simulink model "TxArray"  (R2021b)
settings: Solver=FixedStepDiscrete  StartTime=0.0  StopTime=50  FixedStep=0.01  RelTol=1e-3  EnableMultiTasking=on
libraries: raspberrypiNetworklib x4, realtime_pacer_lib x1
settings Model: SnapshotBufferSize=50  PacingRate=1000  Creator=Blade  LastModifiedBy=Blade
settings SolverCC: PositivePriorityOrder=on

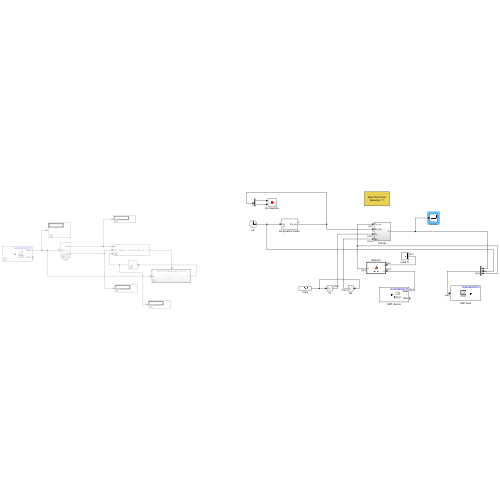
[thumbnail: Simulink's stored preview of the top-level diagram]
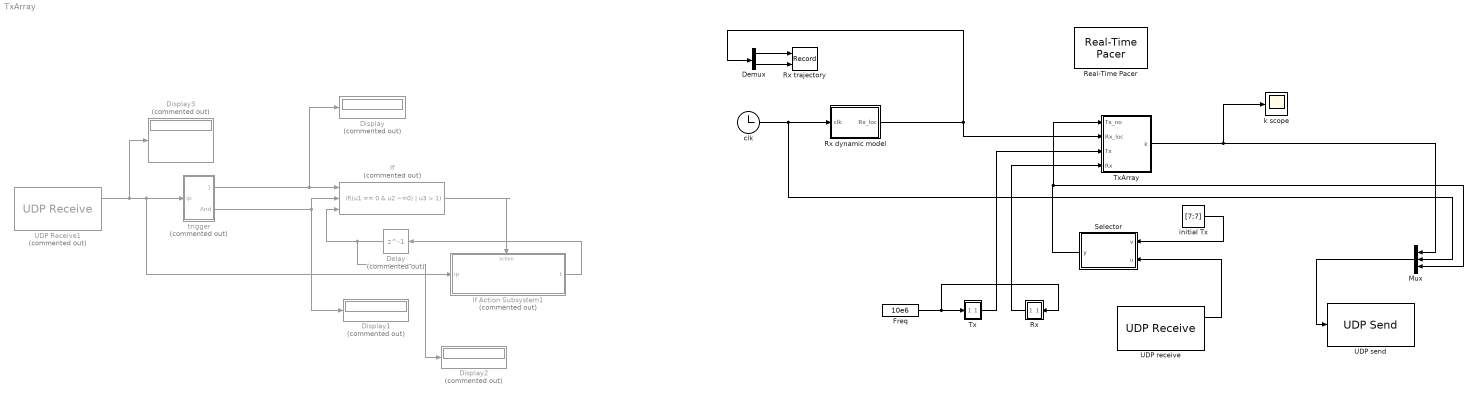
== system TxArray ==
  Delay : Delay  Commented=on  DelayLength=1  InitialCondition=0
  Demux : Demux  Outputs=2
  Display{,1..3} (4 alike) : Display  Commented=on
  Freq : Constant  Value=10e6
  If : If  Commented=on  NumInputs=3  IfExpression=(u1 == 0 & u2 ~=0) | u3 > 1  ShowElse=off
  If Action Subsystem1 : Subsystem  Commented=on  TreatAsAtomicUnit=on
  Mux : Mux  Inputs=3
  Real-Time Pacer : realtime_pacer_lib/Real-Time Pacer  simTimePerRealTime=1
      settings: SourceProductName=Real-Time Pacer
  Rx : Subsystem  mask{dout=1/3*100e-3, phi=0.15, s=800e-6, w=1200e-6, CP=0, SR=0.01}
      mask prompts: dout "out diameter"; phi "fillfact"; s "track spacing"; w "track width"; CP "parasitic capacitance"; SR "source resistance"
      mask TypeOptions dout: Constant1/Value
      mask TypeOptions phi: Constant2/Value
      mask TypeOptions s: Constant3/Value
      mask TypeOptions w: Constant4/Value
      mask TypeOptions CP: Constant6/Value
      mask TypeOptions SR: Constant7/Value
  "Rx dynamic model " : Subsystem  mask{initx=1/2*100e-3*(7+1), inity=1/2*100e-3*(7+1), v_min=[0.01,0.01], v_max=[0.02,0.02]}
      mask prompts: initx "Rx initial x"; inity "Rx initial y"; v_min "Rx min speed"; v_max "Rx max speed"
      mask TypeOptions initx: Delay1/InitialCondition
      mask TypeOptions inity: Delay2/InitialCondition
      mask TypeOptions v_min: Constant/Value
      mask TypeOptions v_max: Constant1/Value
  Rx trajectory : Record  RecordToWorkspace=on  FileSettingsInternal="{\"entries\":[{\"content\":{\"excelSettings\":{\"content\":{},\"type\":\"Streamout.ExcelSettings\"}},\"type\":\"Streamout.FileSettingStorage\",\"uuid\":\"31a4ec05-c512-48d1-876e-5766672d7d43\"}],\"packageUris\":[\"http://schema.mathworks.com/mf0/streamout_blocks/R2020a\"],\"version\":\"1.0\"}"  Layout=[1 1]  SignalsInternal="{\"entries\":[{\"content\":{\"signals\":[{\"content\":{\"blockPath\":[\"TxArray/Rx trajectory\"],\"channel\":[],\"dimensions\":[1],\"domain\":\"TxArray/Rx trajectory\",\"lineColor\":\"#a2142f\",\"plots\":[1],\"port\":1,\"sid\":[\"\"],\"signalID\":51290,\"signalName\":\"Demux:1\"},\"type\":\"RecordBlkView.Signal\",\"uuid\":\"0aae7323-a21c-435c-a499-c26e652a0b80\"},{\"content\":{\"blockPath\":[\"TxArray/Rx trajectory\"],\"channel\":[],\"dimensions\":[1],\"domain\":\"TxArray/Rx trajectory\",\"lineColor\":\"#139fff\",\"plots\":[1],\"port\":2,\"sid\":[\"\"],\"signalID\":51294,\"signalName\":\"Demux:2\"},\"type\":\"RecordBlkView.Signal\",\"uuid\":\"970d65ca-2c0e-4b4c-8729-1a3121c9315b\"}]},\"type\":\"RecordBlkView.InputSignals\",\"uuid\":\"1676dd2b-c950-4d6b-bdb0-46605d271428\"}],\"packageUris\":[\"http://schema.mathworks.com/mf0/streamout_blocks/R2020a\"],\"version\":\"1.0\"}"  VisualizationBindings="{\"xyplotplugin\":{\"info\":[{\"series\":[{\"bindingParametersList\":[{\"parameter\":\"X-Axis\",\"signalID\":51290,\"signalName\":\"Demux:1\"},{\"parameter\":\"Y-Axis\",\"signalID\":51294,\"signalName\":\"Demux:2\"}],\"seriesID\":44186}],\"subplotID\":1}]}}"  CompatibilityTag=XY
  Selector : MATLAB Function  TreatAsAtomicUnit=on
  Tx : Subsystem  mask{dout=100e-3, phi=0.25, s=3*2500e-6, w=2500e-6, CP=0, SR=0.01}
      mask prompts: dout "out diameter"; phi "fillfact"; s "track spacing"; w "track width"; CP "parasitic capacitance"; SR "source resistance"
      mask TypeOptions dout: Constant1/Value
      mask TypeOptions phi: Constant2/Value
      mask TypeOptions s: Constant3/Value
      mask TypeOptions w: Constant4/Value
      mask TypeOptions CP: Constant6/Value
      mask TypeOptions SR: Constant7/Value
  TxArray : Subsystem
  UDP Receive1 : raspberrypiNetworklib/UDP Receive  Commented=on  localURL='0.0.0.0'  localPort=1000  remoteURL='0.0.0.0'  remotePort=-1  recvBufferSize=8192  signalDatatype=double  dims=4  isVarSize=off  showBlockingTime=off  blockingTime=0  sampletime=-1  blockPlatform=Raspberry Pi
      settings: SourceProductBaseCode=RASPPI
  UDP receive : raspberrypiNetworklib/UDP Receive  localURL='0.0.0.0'  localPort=2000  remoteURL='0.0.0.0'  remotePort=-1  recvBufferSize=8192  signalDatatype=double  dims=2  isVarSize=off  showBlockingTime=off  blockingTime=0  sampletime=-1  blockPlatform=Raspberry Pi
      settings: SourceProductBaseCode=RASPPI
  UDP send : raspberrypiNetworklib/UDP Send  remoteURL='172.20.10.3'  remotePort=1000  localURL='0.0.0.0'  localPortSource=Automatically determine  localPort=-1  sampletime=-1  blockPlatform=Raspberry Pi  separateLengthPort=0
      settings: SourceProductBaseCode=RASPPI
  clk : Clock
  initial Tx : Constant  Value=[7;7]  VectorParams1D=off
  k scope : Scope
  trigger : Subsystem  Commented=on
  wires:
  Rx/1(Out1) -> TxArray/4(Rx)
  "Rx dynamic model "/1(Rx_loc) -> TxArray/2(Rx_loc), Demux/1
  Demux/1 -> Rx trajectory/1
  Freq/1 -> Rx/1(In1), Tx/1(In1)
  Demux/2 -> Rx trajectory/2
  Tx/1(Out1) -> TxArray/3(Tx)
  clk/1 -> Mux/2, "Rx dynamic model "/1(clk)
  TxArray/1(k) -> k scope/1, Mux/1
  Selector/1(y) -> Mux/3, TxArray/1(Tx_no)
  UDP receive/1 -> Selector/2(u)
  Mux/1 -> UDP send/1
  initial Tx/1 -> Selector/1(v)
  If/1 -> If Action Subsystem1/Action
  If Action Subsystem1/1(t) -> Delay/1
  trigger/1(mod) -> If/1, Display/1
  Delay/1 -> Display2/1, If/3
  trigger/2(And) -> If/2, Display1/1
  UDP Receive1/1 -> Display3/1, If Action Subsystem1/1(ip), trigger/1(ip)

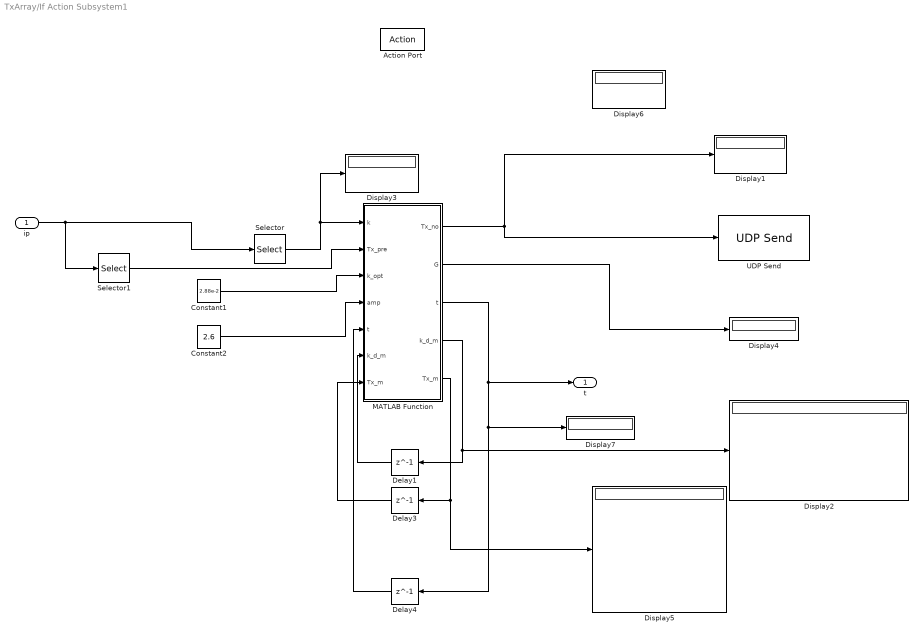
== system TxArray/If Action Subsystem1 ==
  ip : Inport
  Action Port : ActionPort  ActionPortLabel=if((u1 == 0 & u2 ~=0) | u3 > 1)
  Constant1 : Constant  Value=2.88e-2
  Constant2 : Constant  Value=2.6
  Delay1 : Delay  DelayLength=1  InitialCondition=zeros(2,3)
  Delay3 : Delay  DelayLength=1  InitialCondition=zeros(8,2)
  Delay4 : Delay  DelayLength=1  InitialCondition=0
  Display{1..7} (7 alike) : Display
  MATLAB Function : MATLAB Function  TreatAsAtomicUnit=on
  Selector : Selector  InputPortWidth=4  IndexOptions=Index vector (dialog)  Indices=1  OutputSizes=1
  Selector1 : Selector  InputPortWidth=4  IndexOptions=Index vector (dialog)  Indices=[3;4]  OutputSizes=1
  UDP Send : raspberrypiNetworklib/UDP Send  remoteURL='172.20.10.2'  remotePort=2000  localURL='0.0.0.0'  localPortSource=Automatically determine  localPort=-1  sampletime=-1  blockPlatform=Raspberry Pi  separateLengthPort=0
      settings: SourceProductBaseCode=RASPPI
  t : Outport
  wires:
  Delay4/1 -> MATLAB Function/5("t ")
  Constant2/1 -> MATLAB Function/4(amp)
  ip/1 -> Selector1/1, Selector/1
  Constant1/1 -> MATLAB Function/3(k_opt)
  MATLAB Function/1(Tx_no) -> UDP Send/1, Display1/1
  MATLAB Function/3(t) -> Display7/1, Delay4/1, t/1
  MATLAB Function/4(k_d_m) -> Delay1/1, Display2/1
  MATLAB Function/5(Tx_m) -> Display5/1, Delay3/1
  Selector/1 -> Display3/1, MATLAB Function/1(k)
  Delay1/1 -> MATLAB Function/6("k_d_m ")
  MATLAB Function/2(G) -> Display4/1
  Delay3/1 -> MATLAB Function/7("Tx_m ")
  Selector1/1 -> MATLAB Function/2(Tx_pre)

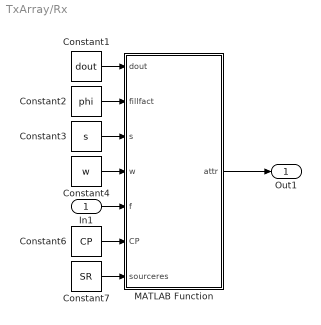
== system TxArray/Rx ==
  In1 : Inport
  Constant1 : Constant  Value=dout
  Constant2 : Constant  Value=phi
  Constant3 : Constant  Value=s
  Constant4 : Constant  Value=w
  Constant6 : Constant  Value=CP
  Constant7 : Constant  Value=SR
  MATLAB Function : MATLAB Function  TreatAsAtomicUnit=on
  Out1 : Outport
  wires:
  MATLAB Function/1(attr) -> Out1/1
  Constant7/1 -> MATLAB Function/7(sourceres)
  Constant1/1 -> MATLAB Function/1(dout)
  Constant2/1 -> MATLAB Function/2(fillfact)
  Constant3/1 -> MATLAB Function/3(s)
  Constant4/1 -> MATLAB Function/4(w)
  In1/1 -> MATLAB Function/5(f)
  Constant6/1 -> MATLAB Function/6(CP)

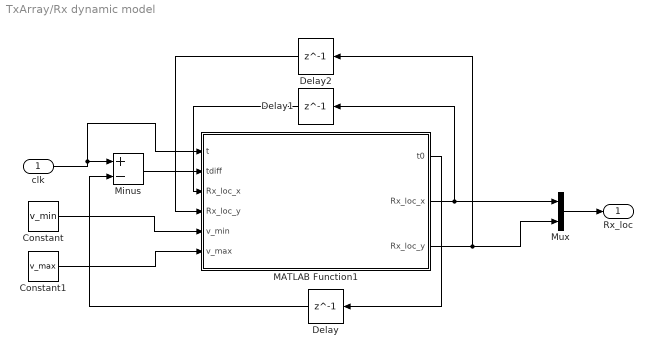
== system TxArray/Rx dynamic model  ==
  clk : Inport
  Constant : Constant  Value=v_min  VectorParams1D=off
  Constant1 : Constant  Value=v_max  VectorParams1D=off
  Delay : Delay  DelayLength=1  InitialCondition=0
  Delay1 : Delay  DelayLength=1  InitialCondition=initx
  Delay2 : Delay  DelayLength=1  InitialCondition=inity
  MATLAB Function1 : MATLAB Function  TreatAsAtomicUnit=on
  Minus : Sum  Inputs=+-
  Mux : Mux  Inputs=2
  Rx_loc : Outport
  wires:
  MATLAB Function1/3(Rx_loc_y) -> Delay2/1, Mux/2
  Delay/1 -> Minus/2
  clk/1 -> MATLAB Function1/1(t), Minus/1
  Delay2/1 -> MATLAB Function1/4("Rx_loc_y ")
  MATLAB Function1/1(t0) -> Delay/1
  Minus/1 -> MATLAB Function1/2(tdiff)
  Delay1/1 -> MATLAB Function1/3("Rx_loc_x ")
  MATLAB Function1/2(Rx_loc_x) -> Delay1/1, Mux/1
  Mux/1 -> Rx_loc/1
  Constant/1 -> MATLAB Function1/5(v_min)
  Constant1/1 -> MATLAB Function1/6(v_max)

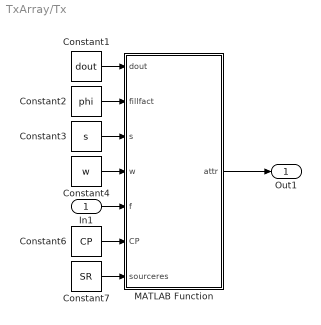
== system TxArray/Tx ==
  In1 : Inport
  Constant1 : Constant  Value=dout
  Constant2 : Constant  Value=phi
  Constant3 : Constant  Value=s
  Constant4 : Constant  Value=w
  Constant6 : Constant  Value=CP
  Constant7 : Constant  Value=SR
  MATLAB Function : MATLAB Function  TreatAsAtomicUnit=on
  Out1 : Outport
  wires:
  MATLAB Function/1(attr) -> Out1/1
  Constant7/1 -> MATLAB Function/7(sourceres)
  Constant1/1 -> MATLAB Function/1(dout)
  Constant2/1 -> MATLAB Function/2(fillfact)
  Constant3/1 -> MATLAB Function/3(s)
  Constant4/1 -> MATLAB Function/4(w)
  In1/1 -> MATLAB Function/5(f)
  Constant6/1 -> MATLAB Function/6(CP)

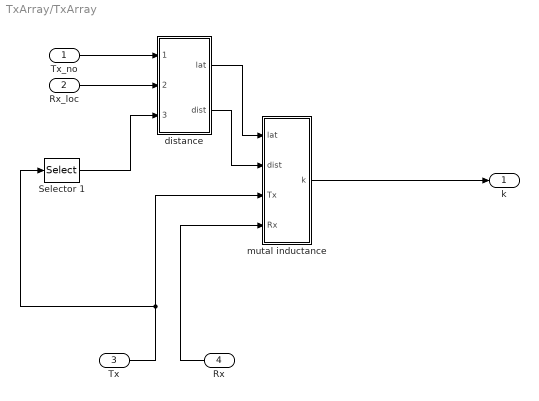
== system TxArray/TxArray ==
  Tx_no : Inport
  Rx_loc : Inport  Port=2
  Tx : Inport  Port=3
  Rx : Inport  Port=4
  " mutal inductance" : Subsystem
  Selector 1 : Selector  InputPortWidth=14  IndexOptions=Index vector (dialog)  Indices=1  OutputSizes=1
  distance : Subsystem
  k : Outport
  wires:
  Tx/1 -> Selector 1/1, " mutal inductance"/3(Tx)
  distance/1(lat) -> " mutal inductance"/1(lat)
  Rx/1 -> " mutal inductance"/4(Rx)
  Tx_no/1 -> distance/1(Tx_no)
  Rx_loc/1 -> distance/2(Rx_loc)
  Selector 1/1 -> distance/3(Tx_dia)
  " mutal inductance"/1(k) -> k/1
  distance/2(dist) -> " mutal inductance"/2(dist)

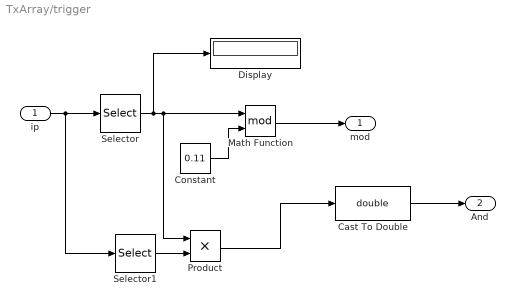
== system TxArray/trigger ==
  ip : Inport
  Cast To Double : DataTypeConversion  OutDataTypeStr=double
  Constant : Constant  Value=0.11
  Display : Display
  Math Function : Math  Operator=mod  SaturateOnIntegerOverflow=on
  Product : Product
  Selector : Selector  InputPortWidth=4  IndexOptions=Index vector (dialog)  Indices=2  OutputSizes=1
  Selector1 : Selector  InputPortWidth=4  IndexOptions=Index vector (dialog)  Indices=1  OutputSizes=1
  mod : Outport
  And : Outport  Port=2
  wires:
  Constant/1 -> Math Function/2
  Selector/1 -> Display/1, Product/1, Math Function/1
  ip/1 -> Selector1/1, Selector/1
  Math Function/1 -> mod/1
  Product/1 -> Cast To Double/1
  Selector1/1 -> Product/2
  Cast To Double/1 -> And/1

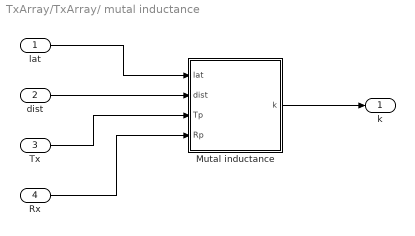
== system TxArray/TxArray/ mutal inductance ==
  lat : Inport
  dist : Inport  Port=2
  Tx : Inport  Port=3
  Rx : Inport  Port=4
  Mutal inductance : MATLAB Function  TreatAsAtomicUnit=on
  k : Outport
  wires:
  lat/1 -> Mutal inductance/1(lat)
  dist/1 -> Mutal inductance/2(dist)
  Tx/1 -> Mutal inductance/3(Tp)
  Rx/1 -> Mutal inductance/4(Rp)
  Mutal inductance/1(k) -> k/1

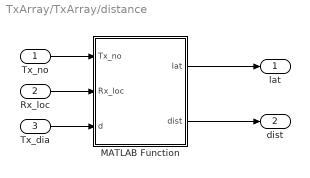
== system TxArray/TxArray/distance ==
  Tx_no : Inport
  Rx_loc : Inport  Port=2
  Tx_dia : Inport  Port=3
  MATLAB Function : MATLAB Function  TreatAsAtomicUnit=on
  lat : Outport
  dist : Outport  Port=2
  wires:
  Tx_dia/1 -> MATLAB Function/3(d)
  Tx_no/1 -> MATLAB Function/1(Tx_no)
  Rx_loc/1 -> MATLAB Function/2(Rx_loc)
  MATLAB Function/1(lat) -> lat/1
  MATLAB Function/2(dist) -> dist/1

== matlab function TxArray/distance/MATLAB Function ==
  data: Tx_no input; Rx_loc input; d input; lat output; dist output
function [lat, dist] = distance(Tx_no, Rx_loc, d)

coder.extrinsic('lat_dist');
coder.extrinsic('vertical_dist');


lat = 0;
dist = 0;

lat = lat_dist(Tx_no, Rx_loc,d);
dist = vertical_dist(Tx_no);
dist = dist + 5e-2;
end

== matlab function TxArray/If Action Subsystem1/MATLAB Function ==
  data: k input; Tx_pre input; Tx_no output; G output; t output; k_opt input; amp input; t input; k_d_m output; k_d_m input; Tx_m input; Tx_m output
function [Tx_no,G,t,k_d_m,Tx_m] = Controller(k,Tx_pre,k_opt,amp,t,k_d_m,Tx_m)

k_diff = abs(k_opt-k)/k_opt;
Tx_pre = Tx_pre';

if t == 0
   

    t = t+1;
    k_d_m(1,:)  = [k_diff,Tx_pre];
    k_d_m(2,:)  = [k_diff,Tx_pre];

    
else

    if k_diff < k_d_m(2,1)

       k_d_m(2,:)  = [k_diff,Tx_pre];

    end

end

G = round(amp*k_d_m(1,1));  
Tx_fix = k_d_m(1,2:3)';

if t < 10
    if t < 9

        dir_att = [-1,-1; -1,0; 0,-1; 1,1; 1,0; 0,1; 1,-1; -1,1];
        
        
        Tx_no =G*dir_att(t,:)'+Tx_fix;
    
        Tx_m (t,:) = Tx_no;

    else

         Tx_no = Tx_fix; % back to centre

    end

    t =t+1;

else
    
    
    Tx_no = k_d_m(2,2:3)';

    t =0;
   
 
end

== matlab function TxArray/ mutal inductance/Mutal inductance ==
  data: lat input; dist input; Tp input; Rp input; k output
function  k = solenoid_MI(lat,dist,Tp,Rp)


coder.extrinsic('MI');

% M = 0;
k = 0;

[~,k] = MI(lat,dist,Tp,Rp);

if k < 0
    k = 0;
end

end

== matlab function TxArray/Tx/MATLAB Function ==
  data: dout input; attr output; fillfact input; s input; w input; f input; CP input; sourceres input
function attr = PCBPhySim(dout,fillfact,s,w,f,CP,sourceres)


y = PCBCoil(dout,fillfact,s,w,f,CP,'square',sourceres);

attr = [y.dout,
    y.din,
    y.fillfact,
    y.w,
    y.s,
    y.n,
    y.L,
    y.Rs,
    y.Q,
    y.C,
    y.CP,
    y.coilZ,
    y.fSRF
    y.f];

== matlab function TxArray/Selector ==
  data: v input; u input; y output
function y = select(v, u)
if u==0

    y = v;
else 
    y = u;
end

== matlab function TxArray/Rx/MATLAB Function ==
  data: dout input; attr output; fillfact input; s input; w input; f input; CP input; sourceres input
function attr = PCBPhySim(dout,fillfact,s,w,f,CP,sourceres)


y = PCBCoil(dout,fillfact,s,w,f,CP,'square',sourceres);

attr = [y.dout,
    y.din,
    y.fillfact,
    y.w,
    y.s,
    y.n,
    y.L,
    y.Rs,
    y.Q,
    y.C,
    y.CP,
    y.coilZ,
    y.fSRF
    y.f];

== matlab function TxArray/Rx dynamic model /MATLAB Function1 ==
  data: t input; tdiff input; t0 output; Rx_loc_x output; Rx_loc_x input; Rx_loc_y input; Rx_loc_y output; v_min input; v_max input
function [t0, Rx_loc_x, Rx_loc_y] = dynamic_on_TxArray(t, tdiff, Rx_loc_x, Rx_loc_y, v_min, v_max)
% if t>=0 && t < 8
%     tdiff = 0;
% elseif t>=10 && t < 19
%     tdiff = 0;
% elseif t>=20 && t < 29
%     tdiff = 0;
% elseif t>=30 && t < 39
%     tdiff = 0;   
% elseif t>=40 && t < 49
%     tdiff = 0;
% elseif t>=50 && t < 59
%     tdiff = 0;
% elseif t>=60 && t < 69
%     tdiff = 0;
% elseif t>=70 && t < 79
%     tdiff = 0;
% elseif t>=80 && t < 89
%     tdiff = 0;
% elseif t>=90 && t < 99
%     tdiff = 0;
% end

% if t>=40 
%      tdiff = 0;
% end

d = 0;
Rx_loc = [Rx_loc_x,Rx_loc_y];
coder.extrinsic('dynamic');
Rx_loc = dynamic(tdiff,Rx_loc,v_min,v_max);
Rx_loc_x = 0;
Rx_loc_y = 0;
Rx_loc_x = Rx_loc(1);
Rx_loc_y = Rx_loc(2);

t0 = t;
